simulink model "impulsiveThruster"  (R2023a)
settings: Solver=ode4  StartTime=0.0  StopTime=10.0  FixedStep=dt  RelTol=1e-3
undefined symbols (not defined in the file): dt
settings Model: Creator=ndelurgio  LastModifiedBy=ndelurgio

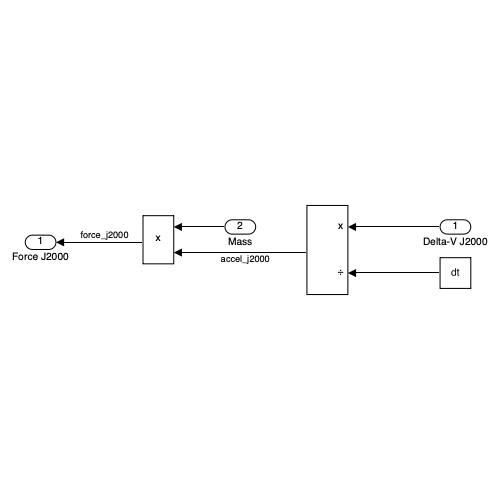
[thumbnail: Simulink's stored preview of the top-level diagram]
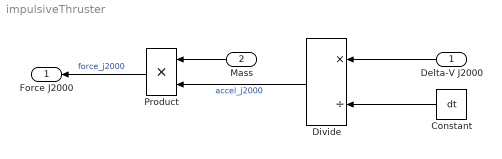
== system impulsiveThruster ==
  Delta-V J2000 : Inport  PortDimensions=3
  Mass : Inport  Port=2
  Constant : Constant  Value=dt
  Divide : Product  Inputs=*/
  Product : Product
  Force J2000 : Outport  PortDimensions=3
  wires:
  Delta-V J2000/1 -> Divide/1
  Constant/1 -> Divide/2
  Divide/1 -> Product/2  "accel_j2000"
  Mass/1 -> Product/1
  Product/1 -> Force J2000/1  "force_j2000"
